simulink model "LateralControllers"  (R2022a)
settings: Solver=VariableStepAuto  StartTime=0.0  StopTime=10.0  RelTol=1e-3
model workspace (MAT data in the model file):
  K = [2.51632988536 0.393907730554 2.24903461301 0.177004257907 -4.17656095855]
  LateralControllers_FeedbackGainLQR = Simulink.Parameter
  LateralControllers_FeedbackGainLQR.Value = [2.51632988536 0.393907730554 2.24903461301 0.177004257907]
  LateralControllers_FeedbackGainLQR.Description = 'LQR feedback gain [K_e1, K_de1, K_e2, K_de2, K_int]'
  LateralControllers_FeedbackGainLQR.DataType = 'double'
  LateralControllers_FeedbackGainLQR.Complexity = 'real'
  LateralControllers_FeedbackGainLQR.Dimensions = [1 4]
  car.m = 1465
  car.Iz = 1600
  car.lf = 1.85
  car.lr = 2.43
  car.Caf = 80000
  car.Car = 80000
settings Model: Creator=krisz  LastModifiedBy=krisz

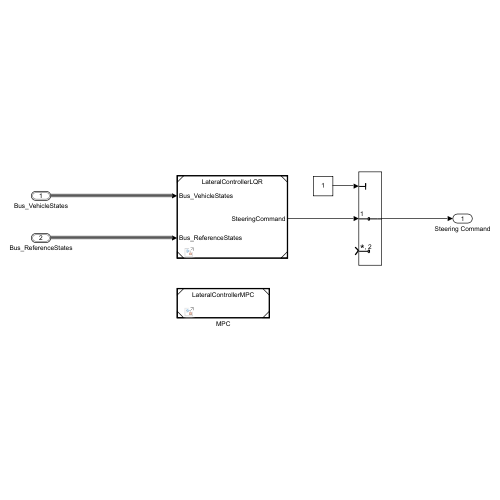
[thumbnail: Simulink's stored preview of the top-level diagram]
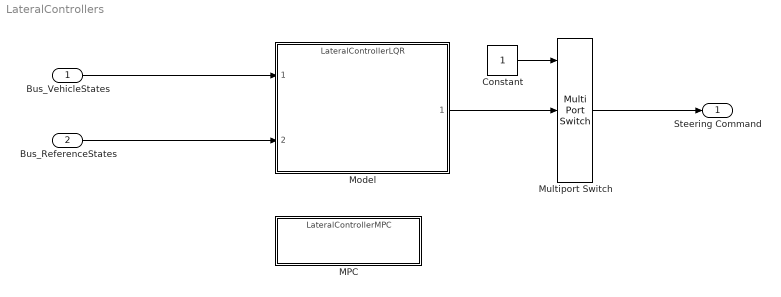
== system LateralControllers ==
  Bus_VehicleStates : Inport  OutDataTypeStr=Bus: bus_VehicleStates
  Bus_ReferenceStates : Inport  Port=2  OutDataTypeStr=Bus: bus_ReferenceStates
  Constant : Constant
  MPC : ModelReference  ModelNameDialog=LateralControllerMPC.slx  SimulationMode=Normal  ModelReferenceVersion=1.0
  Model : ModelReference  ModelNameDialog=LateralControllerLQR.slx  SimulationMode=Normal  ModelReferenceVersion=1.25
  Multiport Switch : MultiPortSwitch  Inputs=2  SaturateOnIntegerOverflow=off  InputSameDT=off
  Steering Command : Outport
  wires:
  Multiport Switch/1 -> Steering Command/1
  Model/1 -> Multiport Switch/2
  Constant/1 -> Multiport Switch/1
  Bus_ReferenceStates/1 -> Model/2
  Bus_VehicleStates/1 -> Model/1
